simulink model "RoboticArmGeneral2DOF_standalonemodel"  (R2022a)
settings: Solver=VariableStepAuto  StartTime=0.0  StopTime=10.0  RelTol=1e-3
undefined symbols (not defined in the file or in its folder): armAttachOffset, smiData, X, Y, Z
libraries: nesl_utility x113, sm_lib x35
(part 2 of 2)

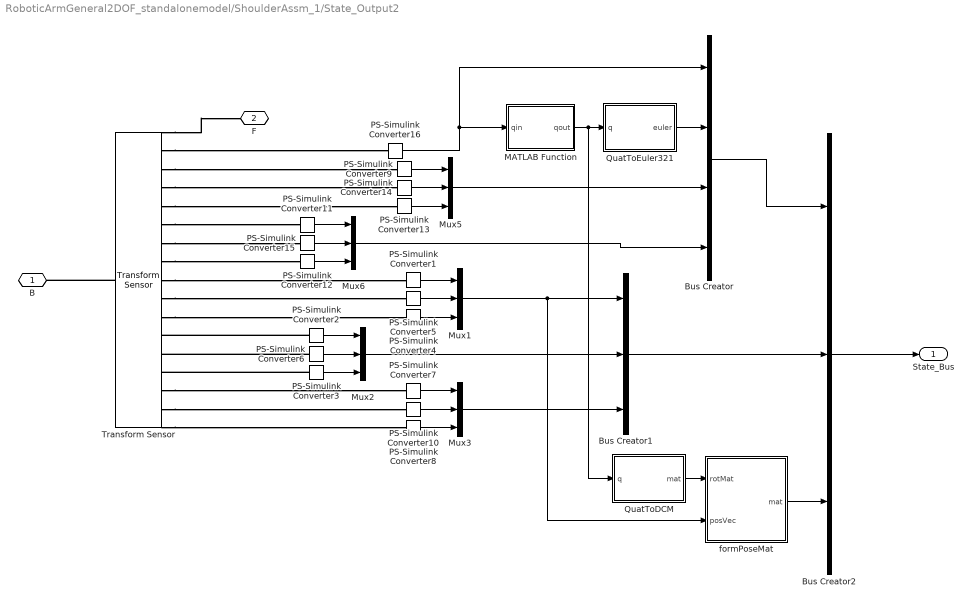
== system RoboticArmGeneral2DOF_standalonemodel/ShoulderAssm_1/State_Output2 ==
  Bus Creator : BusCreator  Inputs=4  OutDataTypeStr=Bus: RotStateBus
      settings: InheritFromInputs=off
  Bus Creator1 : BusCreator  Inputs=3  OutDataTypeStr=Bus: TransStateBus
      settings: InheritFromInputs=off
  Bus Creator2 : BusCreator  Inputs=3  OutDataTypeStr=Bus: StateBus
      settings: InheritFromInputs=off
  MATLAB Function : MATLAB Function  TreatAsAtomicUnit=on
  Mux{1..3,5..6} (5 alike) : Mux  Inputs=3
  PS-Simulink Converter{1..16} (16 alike) : nesl_utility/PS-Simulink Converter  PhysicalDomain=network_engine_domain  SubClassName=ps_output  LeftPortType=input  RightPortType=output  PseudoPeriodic=off  Frequencies=[]  VectorFormat=1-D array  Unit=inherit  AffineConversion=off
      settings: SourceProductBaseCode=SS,PW,VE
  QuatToDCM : MATLAB Function  TreatAsAtomicUnit=on
  QuatToEuler321 : MATLAB Function  TreatAsAtomicUnit=on
  Transform Sensor : sm_lib/Frames and Transforms/Transform Sensor  MeasurementFrame=World  SenseAngle=off  SenseAxis=off  SenseAngle1=off  SenseAngle2=off  SenseAngle3=off  SenseQ=on  SenseR=off  SenseOmegaX=on  SenseOmegaY=on  SenseOmegaZ=on  SenseOmega1=off  SenseOmega2=off  SenseOmega3=off  SenseQDot=off  SenseRDot=off  SenseAlphaX=on  SenseAlphaY=on  SenseAlphaZ=on  SenseAlpha1=off  SenseAlpha2=off  SenseAlpha3=off  SenseQDDot=off  SenseRDDot=off  SenseX=on  SenseY=on  SenseZ=on  SenseRad=off  SenseAzim=off  SenseDist=off  SenseInc=off  SenseXDot=on  SenseYDot=on  SenseZDot=on  SenseRadDot=off  SenseAzimDot=off  SenseDistDot=off  SenseIncDot=off  SenseXDDot=on  SenseYDDot=on  SenseZDDot=on  SenseRadDDot=off  SenseAzimDDot=off  SenseDistDDot=off  SenseIncDDot=off
  formPoseMat : MATLAB Function  TreatAsAtomicUnit=on
  B : PMIOPort  Side=Left
  F : PMIOPort  Port=2  Side=Right
  State_Bus : Outport
  wires:
  formPoseMat/1(mat) -> Bus Creator2/3
  QuatToDCM/1(mat) -> formPoseMat/1(rotMat)
  MATLAB Function/1(qout) -> QuatToEuler321/1(q), QuatToDCM/1(q)
  Bus Creator2/1 -> State_Bus/1
  Bus Creator1/1 -> Bus Creator2/2
  Bus Creator/1 -> Bus Creator2/1
  QuatToEuler321/1(euler) -> Bus Creator/2
  PS-Simulink Converter16/1 -> MATLAB Function/1(qin), Bus Creator/1
  PS-Simulink Converter11/1 -> Mux6/1
  Mux6/1 -> Bus Creator/4
  PS-Simulink Converter12/1 -> Mux6/3
  PS-Simulink Converter15/1 -> Mux6/2
  Mux5/1 -> Bus Creator/3
  PS-Simulink Converter13/1 -> Mux5/3
  PS-Simulink Converter14/1 -> Mux5/2
  PS-Simulink Converter9/1 -> Mux5/1
  Mux3/1 -> Bus Creator1/3
  Mux1/1 -> Bus Creator1/1, formPoseMat/2(posVec)
  Mux2/1 -> Bus Creator1/2
  PS-Simulink Converter7/1 -> Mux3/1
  PS-Simulink Converter8/1 -> Mux3/3
  PS-Simulink Converter10/1 -> Mux3/2
  PS-Simulink Converter2/1 -> Mux2/1
  PS-Simulink Converter6/1 -> Mux2/2
  PS-Simulink Converter3/1 -> Mux2/3
  PS-Simulink Converter1/1 -> Mux1/1
  PS-Simulink Converter5/1 -> Mux1/2
  PS-Simulink Converter4/1 -> Mux1/3
  connections:
  Transform Sensor/RConn2 -- PS-Simulink Converter16/LConn1
  Transform Sensor/RConn6 -- PS-Simulink Converter11/LConn1
  Transform Sensor/RConn7 -- PS-Simulink Converter15/LConn1
  Transform Sensor/RConn3 -- PS-Simulink Converter9/LConn1
  Transform Sensor/RConn4 -- PS-Simulink Converter14/LConn1
  Transform Sensor/RConn5 -- PS-Simulink Converter13/LConn1
  Transform Sensor/RConn8 -- PS-Simulink Converter12/LConn1
  Transform Sensor/RConn16 -- PS-Simulink Converter10/LConn1
  Transform Sensor/RConn15 -- PS-Simulink Converter7/LConn1
  Transform Sensor/RConn17 -- PS-Simulink Converter8/LConn1
  PS-Simulink Converter2/LConn1 -- Transform Sensor/RConn12
  PS-Simulink Converter6/LConn1 -- Transform Sensor/RConn13
  PS-Simulink Converter3/LConn1 -- Transform Sensor/RConn14
  Transform Sensor/RConn11 -- PS-Simulink Converter4/LConn1
  Transform Sensor/RConn10 -- PS-Simulink Converter5/LConn1
  Transform Sensor/RConn9 -- PS-Simulink Converter1/LConn1
  Transform Sensor/RConn1 -- F/RConn1
  Transform Sensor/LConn1 -- B/RConn1

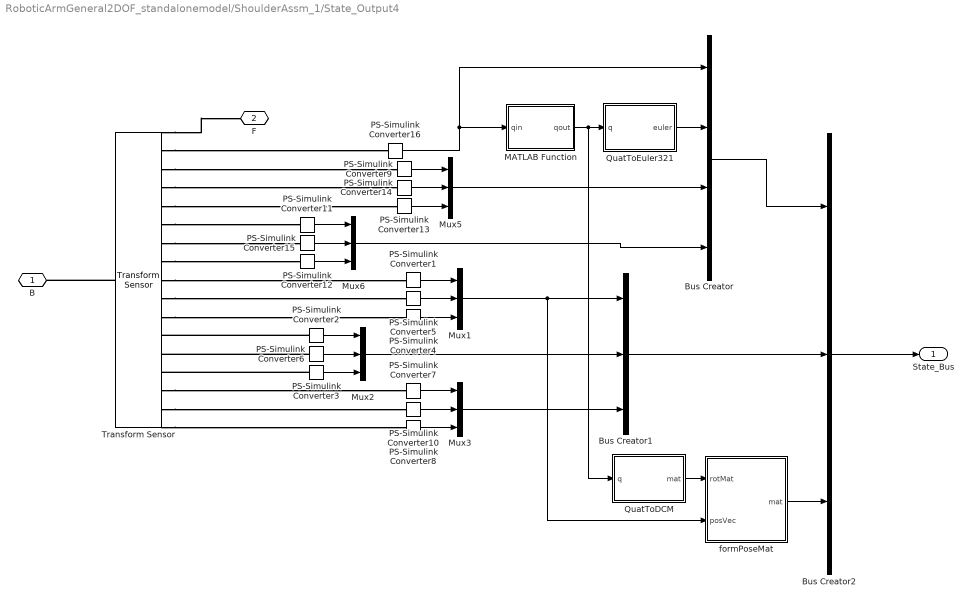
== system RoboticArmGeneral2DOF_standalonemodel/ShoulderAssm_1/State_Output4 ==
  Bus Creator : BusCreator  Inputs=4  OutDataTypeStr=Bus: RotStateBus
      settings: InheritFromInputs=off
  Bus Creator1 : BusCreator  Inputs=3  OutDataTypeStr=Bus: TransStateBus
      settings: InheritFromInputs=off
  Bus Creator2 : BusCreator  Inputs=3  OutDataTypeStr=Bus: StateBus
      settings: InheritFromInputs=off
  MATLAB Function : MATLAB Function  TreatAsAtomicUnit=on
  Mux{1..3,5..6} (5 alike) : Mux  Inputs=3
  PS-Simulink Converter{1..16} (16 alike) : nesl_utility/PS-Simulink Converter  PhysicalDomain=network_engine_domain  SubClassName=ps_output  LeftPortType=input  RightPortType=output  PseudoPeriodic=off  Frequencies=[]  VectorFormat=1-D array  Unit=inherit  AffineConversion=off
      settings: SourceProductBaseCode=SS,PW,VE
  QuatToDCM : MATLAB Function  TreatAsAtomicUnit=on
  QuatToEuler321 : MATLAB Function  TreatAsAtomicUnit=on
  Transform Sensor : sm_lib/Frames and Transforms/Transform Sensor  MeasurementFrame=World  SenseAngle=off  SenseAxis=off  SenseAngle1=off  SenseAngle2=off  SenseAngle3=off  SenseQ=on  SenseR=off  SenseOmegaX=on  SenseOmegaY=on  SenseOmegaZ=on  SenseOmega1=off  SenseOmega2=off  SenseOmega3=off  SenseQDot=off  SenseRDot=off  SenseAlphaX=on  SenseAlphaY=on  SenseAlphaZ=on  SenseAlpha1=off  SenseAlpha2=off  SenseAlpha3=off  SenseQDDot=off  SenseRDDot=off  SenseX=on  SenseY=on  SenseZ=on  SenseRad=off  SenseAzim=off  SenseDist=off  SenseInc=off  SenseXDot=on  SenseYDot=on  SenseZDot=on  SenseRadDot=off  SenseAzimDot=off  SenseDistDot=off  SenseIncDot=off  SenseXDDot=on  SenseYDDot=on  SenseZDDot=on  SenseRadDDot=off  SenseAzimDDot=off  SenseDistDDot=off  SenseIncDDot=off
  formPoseMat : MATLAB Function  TreatAsAtomicUnit=on
  B : PMIOPort  Side=Left
  F : PMIOPort  Port=2  Side=Right
  State_Bus : Outport
  wires:
  formPoseMat/1(mat) -> Bus Creator2/3
  QuatToDCM/1(mat) -> formPoseMat/1(rotMat)
  MATLAB Function/1(qout) -> QuatToEuler321/1(q), QuatToDCM/1(q)
  Bus Creator2/1 -> State_Bus/1
  Bus Creator1/1 -> Bus Creator2/2
  Bus Creator/1 -> Bus Creator2/1
  QuatToEuler321/1(euler) -> Bus Creator/2
  PS-Simulink Converter16/1 -> MATLAB Function/1(qin), Bus Creator/1
  PS-Simulink Converter11/1 -> Mux6/1
  Mux6/1 -> Bus Creator/4
  PS-Simulink Converter12/1 -> Mux6/3
  PS-Simulink Converter15/1 -> Mux6/2
  Mux5/1 -> Bus Creator/3
  PS-Simulink Converter13/1 -> Mux5/3
  PS-Simulink Converter14/1 -> Mux5/2
  PS-Simulink Converter9/1 -> Mux5/1
  Mux3/1 -> Bus Creator1/3
  Mux1/1 -> Bus Creator1/1, formPoseMat/2(posVec)
  Mux2/1 -> Bus Creator1/2
  PS-Simulink Converter7/1 -> Mux3/1
  PS-Simulink Converter8/1 -> Mux3/3
  PS-Simulink Converter10/1 -> Mux3/2
  PS-Simulink Converter2/1 -> Mux2/1
  PS-Simulink Converter6/1 -> Mux2/2
  PS-Simulink Converter3/1 -> Mux2/3
  PS-Simulink Converter1/1 -> Mux1/1
  PS-Simulink Converter5/1 -> Mux1/2
  PS-Simulink Converter4/1 -> Mux1/3
  connections:
  Transform Sensor/RConn2 -- PS-Simulink Converter16/LConn1
  Transform Sensor/RConn6 -- PS-Simulink Converter11/LConn1
  Transform Sensor/RConn7 -- PS-Simulink Converter15/LConn1
  Transform Sensor/RConn3 -- PS-Simulink Converter9/LConn1
  Transform Sensor/RConn4 -- PS-Simulink Converter14/LConn1
  Transform Sensor/RConn5 -- PS-Simulink Converter13/LConn1
  Transform Sensor/RConn8 -- PS-Simulink Converter12/LConn1
  Transform Sensor/RConn16 -- PS-Simulink Converter10/LConn1
  Transform Sensor/RConn15 -- PS-Simulink Converter7/LConn1
  Transform Sensor/RConn17 -- PS-Simulink Converter8/LConn1
  PS-Simulink Converter2/LConn1 -- Transform Sensor/RConn12
  PS-Simulink Converter6/LConn1 -- Transform Sensor/RConn13
  PS-Simulink Converter3/LConn1 -- Transform Sensor/RConn14
  Transform Sensor/RConn11 -- PS-Simulink Converter4/LConn1
  Transform Sensor/RConn10 -- PS-Simulink Converter5/LConn1
  Transform Sensor/RConn9 -- PS-Simulink Converter1/LConn1
  Transform Sensor/RConn1 -- F/RConn1
  Transform Sensor/LConn1 -- B/RConn1

== matlab function RoboticArmGeneral2DOF_standalonemodel/State_Output1/QuatToEuler321 ==
  data: q input; euler output
function euler  = callQuatToEuler321(q)


[euler] = quatToEuler_321(q);

== matlab function RoboticArmGeneral2DOF_standalonemodel/State_Output1/formPoseMat ==
  data: rotMat input; mat output; posVec input
function mat  = callFormPoseMat(rotMat,posVec)


[mat] = formPoseMat(rotMat,posVec);

== matlab function RoboticArmGeneral2DOF_standalonemodel/State_Output2/MATLAB Function ==
  data: qin input; qout output
function qout = call_quatconj(qin)

qout = zeros(1,4);
qout = quatconj(qin');

== matlab function RoboticArmGeneral2DOF_standalonemodel/State_Output2/QuatToDCM ==
  data: q input; mat output
function mat  = callQuatToDCM(q)

[mat] = quatToDCM(q);

== matlab function RoboticArmGeneral2DOF_standalonemodel/State_Output2/QuatToEuler321 ==
  data: q input; euler output
function euler  = callQuatToEuler321(q)


[euler] = quatToEuler_321(q);

== matlab function RoboticArmGeneral2DOF_standalonemodel/State_Output2/formPoseMat ==
  data: rotMat input; mat output; posVec input
function mat  = callFormPoseMat(rotMat,posVec)


[mat] = formPoseMat(rotMat,posVec);

== matlab function RoboticArmGeneral2DOF_standalonemodel/State_Output3/MATLAB Function ==
  data: qin input; qout output
function qout = call_quatconj(qin)

qout = zeros(1,4);
qout = quatconj(qin');

== matlab function RoboticArmGeneral2DOF_standalonemodel/State_Output3/QuatToDCM ==
  data: q input; mat output
function mat  = callQuatToDCM(q)

[mat] = quatToDCM(q);

== matlab function RoboticArmGeneral2DOF_standalonemodel/State_Output3/QuatToEuler321 ==
  data: q input; euler output
function euler  = callQuatToEuler321(q)


[euler] = quatToEuler_321(q);

== matlab function RoboticArmGeneral2DOF_standalonemodel/State_Output3/formPoseMat ==
  data: rotMat input; mat output; posVec input
function mat  = callFormPoseMat(rotMat,posVec)


[mat] = formPoseMat(rotMat,posVec);

== matlab function RoboticArmGeneral2DOF_standalonemodel/ShoulderAssm_1/State_Output4/MATLAB Function ==
  data: qin input; qout output
function qout = call_quatconj(qin)

qout = zeros(1,4);
qout = quatconj(qin');

== matlab function RoboticArmGeneral2DOF_standalonemodel/ShoulderAssm_1/State_Output4/QuatToDCM ==
  data: q input; mat output
function mat  = callQuatToDCM(q)

[mat] = quatToDCM(q);

== matlab function RoboticArmGeneral2DOF_standalonemodel/ShoulderAssm_1/State_Output4/QuatToEuler321 ==
  data: q input; euler output
function euler  = callQuatToEuler321(q)


[euler] = quatToEuler_321(q);

== matlab function RoboticArmGeneral2DOF_standalonemodel/ShoulderAssm_1/State_Output4/formPoseMat ==
  data: rotMat input; mat output; posVec input
function mat  = callFormPoseMat(rotMat,posVec)


[mat] = formPoseMat(rotMat,posVec);

== matlab function RoboticArmGeneral2DOF_standalonemodel/ShoulderAssm_1/State_Output1/MATLAB Function ==
  data: qin input; qout output
function qout = call_quatconj(qin)

qout = zeros(1,4);
qout = quatconj(qin');

== matlab function RoboticArmGeneral2DOF_standalonemodel/ShoulderAssm_1/State_Output1/QuatToDCM ==
  data: q input; mat output
function mat  = callQuatToDCM(q)

[mat] = quatToDCM(q);

== matlab function RoboticArmGeneral2DOF_standalonemodel/ShoulderAssm_1/State_Output1/QuatToEuler321 ==
  data: q input; euler output
function euler  = callQuatToEuler321(q)


[euler] = quatToEuler_321(q);

== matlab function RoboticArmGeneral2DOF_standalonemodel/ShoulderAssm_1/State_Output1/formPoseMat ==
  data: rotMat input; mat output; posVec input
function mat  = callFormPoseMat(rotMat,posVec)


[mat] = formPoseMat(rotMat,posVec);

== matlab function RoboticArmGeneral2DOF_standalonemodel/ShoulderAssm_1/State_Output2/MATLAB Function ==
  data: qin input; qout output
function qout = call_quatconj(qin)

qout = zeros(1,4);
qout = quatconj(qin');

== matlab function RoboticArmGeneral2DOF_standalonemodel/ShoulderAssm_1/State_Output2/QuatToDCM ==
  data: q input; mat output
function mat  = callQuatToDCM(q)

[mat] = quatToDCM(q);

== matlab function RoboticArmGeneral2DOF_standalonemodel/ShoulderAssm_1/State_Output2/QuatToEuler321 ==
  data: q input; euler output
function euler  = callQuatToEuler321(q)


[euler] = quatToEuler_321(q);

== matlab function RoboticArmGeneral2DOF_standalonemodel/ShoulderAssm_1/State_Output2/formPoseMat ==
  data: rotMat input; mat output; posVec input
function mat  = callFormPoseMat(rotMat,posVec)


[mat] = formPoseMat(rotMat,posVec);

== matlab function RoboticArmGeneral2DOF_standalonemodel/State_Output1/MATLAB Function ==
  data: qin input; qout output
function qout = call_quatconj(qin)

qout = zeros(1,4);
qout = quatconj(qin');

== matlab function RoboticArmGeneral2DOF_standalonemodel/State_Output1/QuatToDCM ==
  data: q input; mat output
function mat  = callQuatToDCM(q)

[mat] = quatToDCM(q);
